simulink library "M160_control_lib"  (Simulink 7.8)
settings: Solver=FixedStepDiscrete  StartTime=0.0  StopTime=10.0  RelTol=1e-3
PreLoadFcn:
  | update_path
undefined symbols (not defined in the file): Egc_tiTEgasFilt, ehooks_medc17flex_devlib_io_block, Fmc_facKFuelMassCorr, Fmc_tiTFuelMassCorr, Itc_rpmEngSpdHyst, Itc_rpmEngSpdMax, Tvc_facDutycyclePIDLimitMax, Tvc_facDutycyclePIDLimitMin, Tvc_facKDutycycle, Tvc_tiTnDutycycle, Tvc_tiTvDutycycle
libraries: simulink x6
(part 1 of 2)
CloseFcn:
  | clear
settings Model: Creator=WLB9FE  LastModifiedBy=Tiger

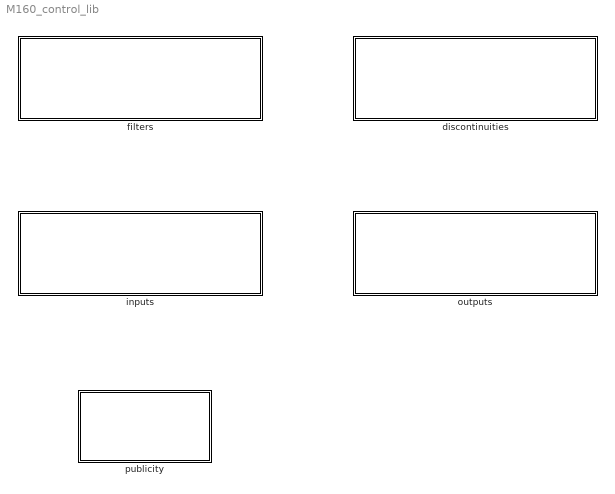
== system M160_control_lib ==
  discontinuities : Subsystem
      mask Display: fprintf('discontinuities')
  filters : Subsystem
      mask Display: fprintf('filters')
  inputs : Subsystem
      mask Display: fprintf('inputs')
  outputs : Subsystem
      mask Display: fprintf('outputs')
  publicity : Subsystem
      mask Description: ETAS
      mask Display: image(imread('ETAS_Logo.jpg'))

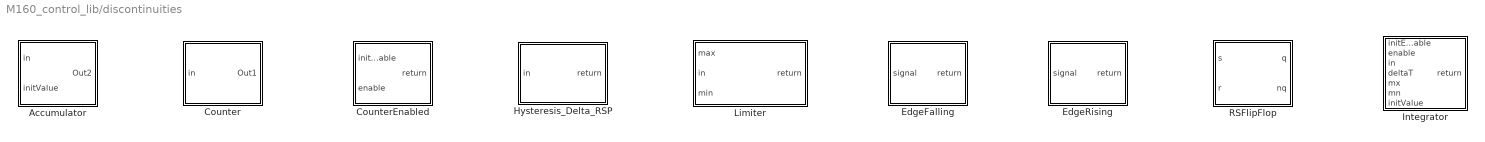
== system M160_control_lib/discontinuities ==
  Accumulator : Subsystem
      mask Description: Accumulator
      mask Display: image(imread('Accumulator.jpg'))
  Counter : Subsystem
      mask Description: Counter
      mask Display: image(imread('Counter.jpg'))
  CounterEnabled : Subsystem
      mask Description: Counter
      mask Display: image(imread('CounterEnabled.jpg'))
  EdgeFalling : Subsystem
      mask Description: EdgeFalling
      mask Display: image(imread('EdgeFalling.jpg'))
  EdgeRising : Subsystem
      mask Description: EdgeRising
      mask Display: image(imread('EdgeRising.jpg'))
  Hysteresis_Delta_RSP : Subsystem
      mask Description: Hysteresis_Delta_RSP
      mask Display: image(imread('HysteresDeltaR.jpg'))
  Integrator : Subsystem
      mask Description: Integrator
      mask Display: image(imread('Integrator.jpg'))
  Limiter : Subsystem
      mask Description: Limiter
      mask Display: image(imread('Limiter.jpg'))
  RSFlipFlop : Subsystem
      mask Description: RSFlipFlop
      mask Display: image(imread('RSFlipFlop.jpg'))

== system M160_control_lib/filters ==
  DT1 : Subsystem
      mask Description: DT1
      mask Display: image(imread('DT1.jpg'))
  DT1_Fcn : Subsystem
      mask Description: DT1_Fcn
      mask Display: image(imread('DT1.jpg'))
  LowpassT : Subsystem
      mask Description: LowpassT
      mask Display: image(imread('LowpassT.jpg'))
  LowpassT_Fcn : Subsystem
      mask Description: LowpassT_Fcn
      mask Display: image(imread('LowpassT.jpg'))
  PID_Limit_AWU : Subsystem
      mask Description: PID_Limit_AWU
      mask Display: image(imread('PID_Limit_AWU.jpg'))
  PID_Limit_AWU_Fcn : Subsystem
      mask Description: PID_Limit_AWU_Fcn
      mask Display: image(imread('PID_Limit_AWU.jpg'))

== system M160_control_lib/inputs ==
  G1_ADC_Input_Receive : Subsystem  LoadFcn=ehooks_medc17flex_devlib_io_block('load');  InitFcn=ehooks_medc17flex_devlib_io_block('init');  StartFcn=ehooks_medc17flex_devlib_io_block('start');  StopFcn=ehooks_medc17flex_devlib_io_block('stop');  ClipboardFcn=ehooks_medc17flex_devlib_io_block('clipboard', 0); % Second argument just needed to indicate null block. See callback handler.  mask{ChannelName=<empty>}
      mask prompts: ChannelName "Channel name"
      mask init:
      | ehooks_medc17flex_devlib_io_block('mask_init');
      settings: AttributesFormatString=Channel name: '%<ChannelName>'  CopyFcn=ehooks_medc17flex_devlib_io_block('copy');  DeleteFcn=ehooks_medc17flex_devlib_io_block('delete');  UndoDeleteFcn=ehooks_medc17flex_devlib_io_block('undo_delete');  ModelCloseFcn=ehooks_medc17flex_devlib_io_block('model_close');  PreSaveFcn=ehooks_medc17flex_devlib_io_block('pre_save');  PostSaveFcn=ehooks_medc17flex_devlib_io_block('post_save');  NameChangeFcn=ehooks_medc17flex_devlib_io_block('name_change');  DestroyFcn=ehooks_medc17flex_devlib_io_block('destroy', 0); % Second argument just needed to indicate null block. See callback handler.  OpenFcn=ehooks_medc17flex_devlib_io_block('open');  CloseFcn=ehooks_medc17flex_devlib_io_block('close');  ParentCloseFcn=ehooks_medc17flex_devlib_io_block('parent_close');  MoveFcn=ehooks_medc17flex_devlib_io_block('move');
      mask StyleString: popup(<empty>|I_A_AN01|I_A_AN02|I_A_AN03|I_A_AN05|I_A_AN06|I_A_AN07|I_A_AN08|I_A_AN10|I_A_AN11|I_A_AN12|I_A_AN13|I_A_AN14|I_A_AN15|I_A_AN16|I_A_AN17|I_A_AN18|I_A_AN19|I_A_AN20|I_A_AN21|I_A_AN23|I_A_AN32|I_A_AN35|I_A_AN36|I_A_AN37|I_A_AN39|I_A_AN100|I_A_AN101|I_A_AN103|I_A_AN104|I_A_AN105|I_A_AN106)
      mask Display: image(imread('Input_Analog.jpg'))
  G1_Digital_Input_Receive : Subsystem  LoadFcn=ehooks_medc17flex_devlib_io_block('load');  InitFcn=ehooks_medc17flex_devlib_io_block('init');  StartFcn=ehooks_medc17flex_devlib_io_block('start');  StopFcn=ehooks_medc17flex_devlib_io_block('stop');  ClipboardFcn=ehooks_medc17flex_devlib_io_block('clipboard', 0); % Second argument just needed to indicate null block. See callback handler.  mask{ChannelName=<empty>}
      mask prompts: ChannelName "Channel name"
      mask init:
      | ehooks_medc17flex_devlib_io_block('mask_init');
      settings: AttributesFormatString=Channel name: '%<ChannelName>'  CopyFcn=ehooks_medc17flex_devlib_io_block('copy');  DeleteFcn=ehooks_medc17flex_devlib_io_block('delete');  UndoDeleteFcn=ehooks_medc17flex_devlib_io_block('undo_delete');  ModelCloseFcn=ehooks_medc17flex_devlib_io_block('model_close');  PreSaveFcn=ehooks_medc17flex_devlib_io_block('pre_save');  PostSaveFcn=ehooks_medc17flex_devlib_io_block('post_save');  NameChangeFcn=ehooks_medc17flex_devlib_io_block('name_change');  DestroyFcn=ehooks_medc17flex_devlib_io_block('destroy', 0); % Second argument just needed to indicate null block. See callback handler.  OpenFcn=ehooks_medc17flex_devlib_io_block('open');  CloseFcn=ehooks_medc17flex_devlib_io_block('close');  ParentCloseFcn=ehooks_medc17flex_devlib_io_block('parent_close');  MoveFcn=ehooks_medc17flex_devlib_io_block('move');
      mask StyleString: popup(<empty>|I_S_T15|I_S_DIG02|I_S_DIG05|I_S_DIG13|I_S_DIG14|I_S_DIG15|I_S_DIG16|I_S_DIG17|I_S_DIG20|I_S_DIG50)
      mask Display: image(imread('Input_Digital.jpg'))
  G1_PWM_Input_Receive : Subsystem  LoadFcn=ehooks_medc17flex_devlib_io_block('load');  InitFcn=ehooks_medc17flex_devlib_io_block('init');  StartFcn=ehooks_medc17flex_devlib_io_block('start');  StopFcn=ehooks_medc17flex_devlib_io_block('stop');  ClipboardFcn=ehooks_medc17flex_devlib_io_block('clipboard', 0); % Second argument just needed to indicate null block. See callback handler.  mask{ChannelName=<empty>}
      mask prompts: ChannelName "Channel name"
      mask init:
      | ehooks_medc17flex_devlib_io_block('mask_init');
      settings: AttributesFormatString=Channel name: '%<ChannelName>'  CopyFcn=ehooks_medc17flex_devlib_io_block('copy');  DeleteFcn=ehooks_medc17flex_devlib_io_block('delete');  UndoDeleteFcn=ehooks_medc17flex_devlib_io_block('undo_delete');  ModelCloseFcn=ehooks_medc17flex_devlib_io_block('model_close');  PreSaveFcn=ehooks_medc17flex_devlib_io_block('pre_save');  PostSaveFcn=ehooks_medc17flex_devlib_io_block('post_save');  NameChangeFcn=ehooks_medc17flex_devlib_io_block('name_change');  DestroyFcn=ehooks_medc17flex_devlib_io_block('destroy', 0); % Second argument just needed to indicate null block. See callback handler.  OpenFcn=ehooks_medc17flex_devlib_io_block('open');  CloseFcn=ehooks_medc17flex_devlib_io_block('close');  ParentCloseFcn=ehooks_medc17flex_devlib_io_block('parent_close');  MoveFcn=ehooks_medc17flex_devlib_io_block('move');
      mask StyleString: popup(<empty>|I_F_DF00|I_F_DF04|I_F_DF06|I_F_DF21|I_F_DF22)
      mask Display: image(imread('Input_Frequency.jpg'))

== system M160_control_lib/outputs ==
  G1_DigOut_Ctrl : Subsystem  LoadFcn=ehooks_medc17flex_devlib_io_block('load');  InitFcn=ehooks_medc17flex_devlib_io_block('init');  StartFcn=ehooks_medc17flex_devlib_io_block('start');  StopFcn=ehooks_medc17flex_devlib_io_block('stop');  ClipboardFcn=ehooks_medc17flex_devlib_io_block('clipboard', 0); % Second argument just needed to indicate null block. See callback handler.  mask{ChannelName=<empty>}
      mask prompts: ChannelName "Channel name"
      mask init:
      | ehooks_medc17flex_devlib_io_block('mask_init');
      settings: AttributesFormatString=Channel name: '%<ChannelName>'  CopyFcn=ehooks_medc17flex_devlib_io_block('copy');  DeleteFcn=ehooks_medc17flex_devlib_io_block('delete');  UndoDeleteFcn=ehooks_medc17flex_devlib_io_block('undo_delete');  ModelCloseFcn=ehooks_medc17flex_devlib_io_block('model_close');  PreSaveFcn=ehooks_medc17flex_devlib_io_block('pre_save');  PostSaveFcn=ehooks_medc17flex_devlib_io_block('post_save');  NameChangeFcn=ehooks_medc17flex_devlib_io_block('name_change');  DestroyFcn=ehooks_medc17flex_devlib_io_block('destroy', 0); % Second argument just needed to indicate null block. See callback handler.  OpenFcn=ehooks_medc17flex_devlib_io_block('open');  CloseFcn=ehooks_medc17flex_devlib_io_block('close');  ParentCloseFcn=ehooks_medc17flex_devlib_io_block('parent_close');  MoveFcn=ehooks_medc17flex_devlib_io_block('move');
      mask StyleString: popup(<empty>|O_S_MRLY|O_S_RL09|O_S_RL14|O_S_RL29|O_S_RL30|O_S_RL31|O_S_RL33|O_S_RL34|O_S_RL35|O_S_RL41|O_S_RL43)
      mask Display: image(imread('Output_Digital.jpg'))
  G1_DigOut_GetError : Subsystem  LoadFcn=ehooks_medc17flex_devlib_io_block('load');  InitFcn=ehooks_medc17flex_devlib_io_block('init');  StartFcn=ehooks_medc17flex_devlib_io_block('start');  StopFcn=ehooks_medc17flex_devlib_io_block('stop');  ClipboardFcn=ehooks_medc17flex_devlib_io_block('clipboard', 0); % Second argument just needed to indicate null block. See callback handler.  mask{ChannelName=<empty>}
      mask prompts: ChannelName "Channel name"
      mask init:
      | ehooks_medc17flex_devlib_io_block('mask_init');
      settings: AttributesFormatString=Channel name: '%<ChannelName>'  CopyFcn=ehooks_medc17flex_devlib_io_block('copy');  DeleteFcn=ehooks_medc17flex_devlib_io_block('delete');  UndoDeleteFcn=ehooks_medc17flex_devlib_io_block('undo_delete');  ModelCloseFcn=ehooks_medc17flex_devlib_io_block('model_close');  PreSaveFcn=ehooks_medc17flex_devlib_io_block('pre_save');  PostSaveFcn=ehooks_medc17flex_devlib_io_block('post_save');  NameChangeFcn=ehooks_medc17flex_devlib_io_block('name_change');  DestroyFcn=ehooks_medc17flex_devlib_io_block('destroy', 0); % Second argument just needed to indicate null block. See callback handler.  OpenFcn=ehooks_medc17flex_devlib_io_block('open');  CloseFcn=ehooks_medc17flex_devlib_io_block('close');  ParentCloseFcn=ehooks_medc17flex_devlib_io_block('parent_close');  MoveFcn=ehooks_medc17flex_devlib_io_block('move');
      mask StyleString: popup(<empty>|O_S_MRLY|O_S_RL09|O_S_RL14|O_S_RL29|O_S_RL30|O_S_RL31|O_S_RL33|O_S_RL34|O_S_RL35|O_S_RL41|O_S_RL43)
      mask Display: image(imread('Output_Digital_Diagnosis.jpg'))
  G1_HbridgeOut_Ctrl : Subsystem  LoadFcn=ehooks_medc17flex_devlib_io_block('load');  InitFcn=ehooks_medc17flex_devlib_io_block('init');  StartFcn=ehooks_medc17flex_devlib_io_block('start');  StopFcn=ehooks_medc17flex_devlib_io_block('stop');  ClipboardFcn=ehooks_medc17flex_devlib_io_block('clipboard', 0); % Second argument just needed to indicate null block. See callback handler.  mask{ChannelName=<empty>}
      mask prompts: ChannelName "Channel name"
      mask init:
      | ehooks_medc17flex_devlib_io_block('mask_init');
      settings: AttributesFormatString=Channel name: '%<ChannelName>'  CopyFcn=ehooks_medc17flex_devlib_io_block('copy');  DeleteFcn=ehooks_medc17flex_devlib_io_block('delete');  UndoDeleteFcn=ehooks_medc17flex_devlib_io_block('undo_delete');  ModelCloseFcn=ehooks_medc17flex_devlib_io_block('model_close');  PreSaveFcn=ehooks_medc17flex_devlib_io_block('pre_save');  PostSaveFcn=ehooks_medc17flex_devlib_io_block('post_save');  NameChangeFcn=ehooks_medc17flex_devlib_io_block('name_change');  DestroyFcn=ehooks_medc17flex_devlib_io_block('destroy', 0); % Second argument just needed to indicate null block. See callback handler.  OpenFcn=ehooks_medc17flex_devlib_io_block('open');  CloseFcn=ehooks_medc17flex_devlib_io_block('close');  ParentCloseFcn=ehooks_medc17flex_devlib_io_block('parent_close');  MoveFcn=ehooks_medc17flex_devlib_io_block('move');
      mask StyleString: popup(<empty>|O_T_DC1|O_T_DC2|O_T_DC3)
      mask Display: image(imread('Output_HBridge.jpg'))
  G1_Hbridge_Get_error : Subsystem  LoadFcn=ehooks_medc17flex_devlib_io_block('load');  InitFcn=ehooks_medc17flex_devlib_io_block('init');  StartFcn=ehooks_medc17flex_devlib_io_block('start');  StopFcn=ehooks_medc17flex_devlib_io_block('stop');  ClipboardFcn=ehooks_medc17flex_devlib_io_block('clipboard', 0); % Second argument just needed to indicate null block. See callback handler.  mask{ChannelName=<empty>}
      mask prompts: ChannelName "Channel name"
      mask init:
      | ehooks_medc17flex_devlib_io_block('mask_init');
      settings: AttributesFormatString=Channel name: '%<ChannelName>'  CopyFcn=ehooks_medc17flex_devlib_io_block('copy');  DeleteFcn=ehooks_medc17flex_devlib_io_block('delete');  UndoDeleteFcn=ehooks_medc17flex_devlib_io_block('undo_delete');  ModelCloseFcn=ehooks_medc17flex_devlib_io_block('model_close');  PreSaveFcn=ehooks_medc17flex_devlib_io_block('pre_save');  PostSaveFcn=ehooks_medc17flex_devlib_io_block('post_save');  NameChangeFcn=ehooks_medc17flex_devlib_io_block('name_change');  DestroyFcn=ehooks_medc17flex_devlib_io_block('destroy', 0); % Second argument just needed to indicate null block. See callback handler.  OpenFcn=ehooks_medc17flex_devlib_io_block('open');  CloseFcn=ehooks_medc17flex_devlib_io_block('close');  ParentCloseFcn=ehooks_medc17flex_devlib_io_block('parent_close');  MoveFcn=ehooks_medc17flex_devlib_io_block('move');
      mask StyleString: popup(<empty>|O_T_DC1|O_T_DC2|O_T_DC3)
      mask Display: image(imread('Output_HBridge_Diagnosis.jpg'))
  G1_IGN_SetParam_for_PFI : Subsystem  LoadFcn=ehooks_medc17flex_devlib_io_block('load');  InitFcn=ehooks_medc17flex_devlib_io_block('init');  StartFcn=ehooks_medc17flex_devlib_io_block('start');  StopFcn=ehooks_medc17flex_devlib_io_block('stop');  ClipboardFcn=ehooks_medc17flex_devlib_io_block('clipboard', 0); % Second argument just needed to indicate null block. See callback handler.  mask{handleName=IGNORED}
      mask prompts: handleName "PlaceHolder_IGNORED"
      mask init:
      | ehooks_medc17flex_devlib_io_block('mask_init');
      settings: CopyFcn=ehooks_medc17flex_devlib_io_block('copy');  DeleteFcn=ehooks_medc17flex_devlib_io_block('delete');  UndoDeleteFcn=ehooks_medc17flex_devlib_io_block('undo_delete');  ModelCloseFcn=ehooks_medc17flex_devlib_io_block('model_close');  PreSaveFcn=ehooks_medc17flex_devlib_io_block('pre_save');  PostSaveFcn=ehooks_medc17flex_devlib_io_block('post_save');  NameChangeFcn=ehooks_medc17flex_devlib_io_block('name_change');  DestroyFcn=ehooks_medc17flex_devlib_io_block('destroy', 0); % Second argument just needed to indicate null block. See callback handler.  OpenFcn=ehooks_medc17flex_devlib_io_block('open');  CloseFcn=ehooks_medc17flex_devlib_io_block('close');  ParentCloseFcn=ehooks_medc17flex_devlib_io_block('parent_close');  MoveFcn=ehooks_medc17flex_devlib_io_block('move');
      mask StyleString: popup(IGNORED)
      mask Display: image(imread('IgnClPfi.jpg'))
  G1_InjVlvPFI_SetParam : Subsystem  LoadFcn=ehooks_medc17flex_devlib_io_block('load');  InitFcn=ehooks_medc17flex_devlib_io_block('init');  StartFcn=ehooks_medc17flex_devlib_io_block('start');  StopFcn=ehooks_medc17flex_devlib_io_block('stop');  ClipboardFcn=ehooks_medc17flex_devlib_io_block('clipboard', 0); % Second argument just needed to indicate null block. See callback handler.  mask{ChannelName=IGNORED}
      mask prompts: ChannelName "PlaceHolder_IGNORED"
      mask init:
      | ehooks_medc17flex_devlib_io_block('mask_init');
      settings: CopyFcn=ehooks_medc17flex_devlib_io_block('copy');  DeleteFcn=ehooks_medc17flex_devlib_io_block('delete');  UndoDeleteFcn=ehooks_medc17flex_devlib_io_block('undo_delete');  ModelCloseFcn=ehooks_medc17flex_devlib_io_block('model_close');  PreSaveFcn=ehooks_medc17flex_devlib_io_block('pre_save');  PostSaveFcn=ehooks_medc17flex_devlib_io_block('post_save');  NameChangeFcn=ehooks_medc17flex_devlib_io_block('name_change');  DestroyFcn=ehooks_medc17flex_devlib_io_block('destroy', 0); % Second argument just needed to indicate null block. See callback handler.  OpenFcn=ehooks_medc17flex_devlib_io_block('open');  CloseFcn=ehooks_medc17flex_devlib_io_block('close');  ParentCloseFcn=ehooks_medc17flex_devlib_io_block('parent_close');  MoveFcn=ehooks_medc17flex_devlib_io_block('move');
      mask StyleString: popup(IGNORED)
      mask Display: image(imread('InjVlvPfi.jpg'))
  G1_Inj_Set_DEVE_forPFI : Subsystem  LoadFcn=ehooks_medc17flex_devlib_io_block('load');  InitFcn=ehooks_medc17flex_devlib_io_block('init');  StartFcn=ehooks_medc17flex_devlib_io_block('start');  StopFcn=ehooks_medc17flex_devlib_io_block('stop');  ClipboardFcn=ehooks_medc17flex_devlib_io_block('clipboard', 0); % Second argument just needed to indicate null block. See callback handler.  mask{ChannelName=IGNORED}
      mask prompts: ChannelName "PlaceHolder_IGNORED"
      mask help: InjVlvDeve
      mask init:
      | ehooks_medc17flex_devlib_io_block('mask_init');
      settings: CopyFcn=ehooks_medc17flex_devlib_io_block('copy');  DeleteFcn=ehooks_medc17flex_devlib_io_block('delete');  UndoDeleteFcn=ehooks_medc17flex_devlib_io_block('undo_delete');  ModelCloseFcn=ehooks_medc17flex_devlib_io_block('model_close');  PreSaveFcn=ehooks_medc17flex_devlib_io_block('pre_save');  PostSaveFcn=ehooks_medc17flex_devlib_io_block('post_save');  NameChangeFcn=ehooks_medc17flex_devlib_io_block('name_change');  DestroyFcn=ehooks_medc17flex_devlib_io_block('destroy', 0); % Second argument just needed to indicate null block. See callback handler.  OpenFcn=ehooks_medc17flex_devlib_io_block('open');  CloseFcn=ehooks_medc17flex_devlib_io_block('close');  ParentCloseFcn=ehooks_medc17flex_devlib_io_block('parent_close');  MoveFcn=ehooks_medc17flex_devlib_io_block('move');
      mask StyleString: popup(IGNORED)
      mask Display: image(imread('InjVlvPfi.jpg'))
  G1_PWM_Output_Ctrl : Subsystem  LoadFcn=ehooks_medc17flex_devlib_io_block('load');  InitFcn=ehooks_medc17flex_devlib_io_block('init');  StartFcn=ehooks_medc17flex_devlib_io_block('start');  StopFcn=ehooks_medc17flex_devlib_io_block('stop');  ClipboardFcn=ehooks_medc17flex_devlib_io_block('clipboard', 0); % Second argument just needed to indicate null block. See callback handler.  mask{ChannelName=<empty>}
      mask prompts: ChannelName "Channel name"
      mask init:
      | ehooks_medc17flex_devlib_io_block('mask_init');
      settings: AttributesFormatString=Channel name: '%<ChannelName>'  CopyFcn=ehooks_medc17flex_devlib_io_block('copy');  DeleteFcn=ehooks_medc17flex_devlib_io_block('delete');  UndoDeleteFcn=ehooks_medc17flex_devlib_io_block('undo_delete');  ModelCloseFcn=ehooks_medc17flex_devlib_io_block('model_close');  PreSaveFcn=ehooks_medc17flex_devlib_io_block('pre_save');  PostSaveFcn=ehooks_medc17flex_devlib_io_block('post_save');  NameChangeFcn=ehooks_medc17flex_devlib_io_block('name_change');  DestroyFcn=ehooks_medc17flex_devlib_io_block('destroy', 0); % Second argument just needed to indicate null block. See callback handler.  OpenFcn=ehooks_medc17flex_devlib_io_block('open');  CloseFcn=ehooks_medc17flex_devlib_io_block('close');  ParentCloseFcn=ehooks_medc17flex_devlib_io_block('parent_close');  MoveFcn=ehooks_medc17flex_devlib_io_block('move');
      mask StyleString: popup(<empty>|O_T_RL10|O_T_RL13|O_T_RL19|O_T_RL20|O_T_RL22|O_T_RL23|O_T_RL25|O_T_RL26|O_T_RL27|O_T_RL28|O_T_RL38|O_T_RL39|O_T_RL40|O_T_RL42|O_T_RL44|O_T_RL45|O_T_RL46|O_T_RL47|O_T_RL48|O_T_RL49|O_T_RL50|O_T_RH02)
      mask Display: image(imread('Output_PWM.jpg'))
  G1_PwmOut_Get_error : Subsystem  LoadFcn=ehooks_medc17flex_devlib_io_block('load');  InitFcn=ehooks_medc17flex_devlib_io_block('init');  StartFcn=ehooks_medc17flex_devlib_io_block('start');  StopFcn=ehooks_medc17flex_devlib_io_block('stop');  ClipboardFcn=ehooks_medc17flex_devlib_io_block('clipboard', 0); % Second argument just needed to indicate null block. See callback handler.  mask{ChannelName=<empty>}
      mask prompts: ChannelName "Channel name"
      mask init:
      | ehooks_medc17flex_devlib_io_block('mask_init');
      settings: AttributesFormatString=Channel name: '%<ChannelName>'  CopyFcn=ehooks_medc17flex_devlib_io_block('copy');  DeleteFcn=ehooks_medc17flex_devlib_io_block('delete');  UndoDeleteFcn=ehooks_medc17flex_devlib_io_block('undo_delete');  ModelCloseFcn=ehooks_medc17flex_devlib_io_block('model_close');  PreSaveFcn=ehooks_medc17flex_devlib_io_block('pre_save');  PostSaveFcn=ehooks_medc17flex_devlib_io_block('post_save');  NameChangeFcn=ehooks_medc17flex_devlib_io_block('name_change');  DestroyFcn=ehooks_medc17flex_devlib_io_block('destroy', 0); % Second argument just needed to indicate null block. See callback handler.  OpenFcn=ehooks_medc17flex_devlib_io_block('open');  CloseFcn=ehooks_medc17flex_devlib_io_block('close');  ParentCloseFcn=ehooks_medc17flex_devlib_io_block('parent_close');  MoveFcn=ehooks_medc17flex_devlib_io_block('move');
      mask StyleString: popup(<empty>|O_T_RL10|O_T_RL13|O_T_RL19|O_T_RL20|O_T_RL22|O_T_RL23|O_T_RL25|O_T_RL26|O_T_RL27|O_T_RL28|O_T_RL38|O_T_RL39|O_T_RL40|O_T_RL42|O_T_RL44|O_T_RL45|O_T_RL46|O_T_RL47|O_T_RL48|O_T_RL49|O_T_RL50|O_T_RH02)
      mask Display: image(imread('Output_PWM_Diagnosis.jpg'))

== system M160_control_lib/publicity ==

== system M160_control_lib/discontinuities/Accumulator ==
  in : Inport
  initValue : Inport  Port=2
  Add : Sum
  MATLAB Function : MATLAB Function  TreatAsAtomicUnit=on
  Switch2 : Switch  Threshold=1
  Unit Delay : UnitDelay  SampleTime=-1
  Out2 : Outport
  wires:
  in/1 -> Add/1, MATLAB Function/1(u)
  Unit Delay/1 -> Add/2
  Switch2/1 -> Out2/1
  initValue/1 -> Switch2/3
  Add/1 -> Switch2/1, Unit Delay/1
  MATLAB Function/1(y) -> Switch2/2

== system M160_control_lib/discontinuities/Counter ==
  in : Inport
  Add1 : Sum
  Constant1 : Constant  OutDataTypeStr=single
  Constant2 : Constant  Value=0  OutDataTypeStr=single
  MATLAB Function : MATLAB Function  TreatAsAtomicUnit=on
  Switch2 : Switch  Threshold=1
  Unit Delay1 : UnitDelay  SampleTime=-1
  Out1 : Outport
  wires:
  Constant1/1 -> Add1/1
  Unit Delay1/1 -> Add1/2
  Switch2/1 -> Out1/1
  Constant2/1 -> Switch2/3
  Add1/1 -> Switch2/1, Unit Delay1/1
  MATLAB Function/1(y) -> Switch2/2
  in/1 -> MATLAB Function/1(u)

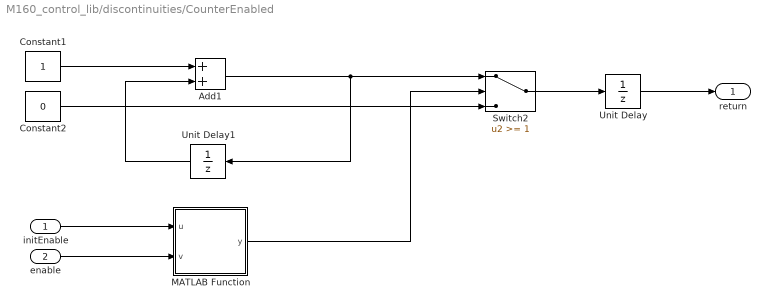
== system M160_control_lib/discontinuities/CounterEnabled ==
  initEnable : Inport
  enable : Inport  Port=2
  Add1 : Sum
  Constant1 : Constant  OutDataTypeStr=single
  Constant2 : Constant  Value=0  OutDataTypeStr=single
  MATLAB Function : MATLAB Function  TreatAsAtomicUnit=on
  Switch2 : Switch  Threshold=1
  Unit Delay : UnitDelay  SampleTime=-1
  Unit Delay1 : UnitDelay  SampleTime=-1
  return : Outport
  wires:
  initEnable/1 -> MATLAB Function/1(u)
  MATLAB Function/1(y) -> Switch2/2
  Add1/1 -> Unit Delay1/1, Switch2/1
  Constant2/1 -> Switch2/3
  Switch2/1 -> Unit Delay/1
  Unit Delay1/1 -> Add1/2
  Constant1/1 -> Add1/1
  enable/1 -> MATLAB Function/2(v)
  Unit Delay/1 -> return/1

== system M160_control_lib/discontinuities/EdgeFalling ==
  signal : Inport
  Detect Decrease : simulink/Logic and Bit Operations/Detect Decrease  vinit=0.0  InputProcessing=Inherited  OutDataTypeStr=boolean
  return : Outport
  wires:
  Detect Decrease/1 -> return/1
  signal/1 -> Detect Decrease/1

== system M160_control_lib/discontinuities/EdgeRising ==
  signal : Inport
  Detect Increase : simulink/Logic and Bit Operations/Detect Increase  vinit=0.0  InputProcessing=Inherited  OutDataTypeStr=boolean
  return : Outport
  wires:
  Detect Increase/1 -> return/1
  signal/1 -> Detect Increase/1

== system M160_control_lib/discontinuities/Hysteresis_Delta_RSP ==
  in : Inport
  Relay : Relay  OnSwitchValue=Itc_rpmEngSpdMax  OffSwitchValue=Itc_rpmEngSpdMax-Itc_rpmEngSpdHyst  OutDataTypeStr=Inherit: Inherit via back propagation
  return : Outport
  wires:
  Relay/1 -> return/1
  in/1 -> Relay/1

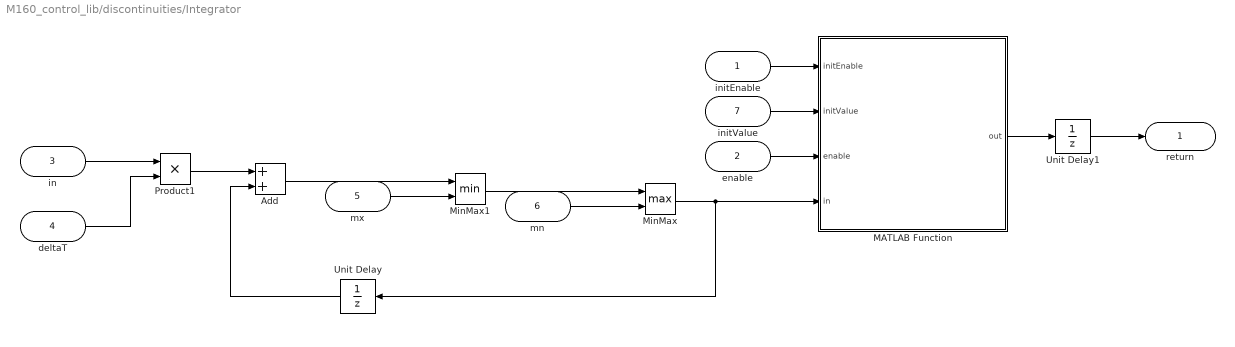
== system M160_control_lib/discontinuities/Integrator ==
  initEnable : Inport
  enable : Inport  Port=2
  in : Inport  Port=3
  deltaT : Inport  Port=4
  mx : Inport  Port=5
  mn : Inport  Port=6
  initValue : Inport  Port=7
  Add : Sum
  MATLAB Function : MATLAB Function  TreatAsAtomicUnit=on
  MinMax : MinMax  Function=max  Inputs=2
  MinMax1 : MinMax  Inputs=2
  Product1 : Product  OutDataTypeStr=Inherit: Same as first input
  Unit Delay : UnitDelay  SampleTime=-1
  Unit Delay1 : UnitDelay  SampleTime=-1
  return : Outport
  wires:
  deltaT/1 -> Product1/2
  in/1 -> Product1/1
  Product1/1 -> Add/1
  Add/1 -> MinMax1/1
  mx/1 -> MinMax1/2
  MinMax1/1 -> MinMax/1
  mn/1 -> MinMax/2
  Unit Delay/1 -> Add/2
  MinMax/1 -> Unit Delay/1, MATLAB Function/4(in)
  MATLAB Function/1(out) -> Unit Delay1/1
  enable/1 -> MATLAB Function/3(enable)
  initValue/1 -> MATLAB Function/2(initValue)
  initEnable/1 -> MATLAB Function/1(initEnable)
  Unit Delay1/1 -> return/1

== system M160_control_lib/discontinuities/Limiter ==
  max : Inport
  in : Inport  Port=2
  min : Inport  Port=3
  Saturation Dynamic : simulink/Discontinuities/Saturation Dynamic  OutMin=[]  OutMax=[]  OutDataTypeStr=Inherit: Same as second input  OutDataType=fixdt(1, 16)  OutScaling=2^-10  DoSatur=off
  return : Outport
  wires:
  max/1 -> Saturation Dynamic/1
  in/1 -> Saturation Dynamic/2
  min/1 -> Saturation Dynamic/3
  Saturation Dynamic/1 -> return/1

== system M160_control_lib/discontinuities/RSFlipFlop ==
  s : Inport
  r : Inport  Port=2
  Gain : Gain  OutDataTypeStr=Inherit: Same as input
  Logical Operator3 : Logic  Operator=NOT  AllPortsSameDT=off  OutDataTypeStr=boolean
  MATLAB Function : MATLAB Function  TreatAsAtomicUnit=on
  Unit Delay : UnitDelay  SampleTime=-1
  q : Outport
  nq : Outport  Port=2
  wires:
  Logical Operator3/1 -> nq/1
  r/1 -> MATLAB Function/1(r)
  s/1 -> MATLAB Function/2(s)
  MATLAB Function/1(q) -> Unit Delay/1
  Gain/1 -> q/1
  Unit Delay/1 -> Logical Operator3/1, Gain/1

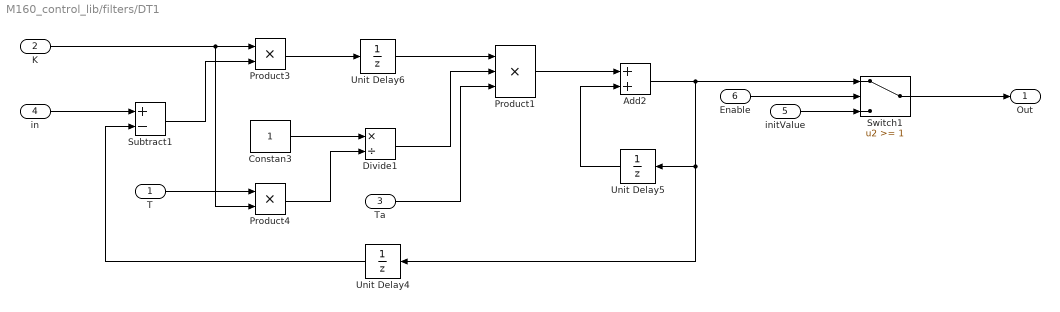
== system M160_control_lib/filters/DT1 ==
  T : Inport
  K : Inport  Port=2
  Ta : Inport  Port=3
  in : Inport  Port=4
  initValue : Inport  Port=5
  Enable : Inport  Port=6
  Add2 : Sum  OutDataTypeStr=Inherit: Same as first input
  Constan3 : Constant  OutDataTypeStr=single
  Divide1 : Product  Inputs=*/  OutDataTypeStr=Inherit: Same as first input
  Product1 : Product  Inputs=3  OutDataTypeStr=Inherit: Same as first input
  Product3 : Product  OutDataTypeStr=Inherit: Same as first input
  Product4 : Product  OutDataTypeStr=Inherit: Same as first input
  Subtract1 : Sum  Inputs=+-
  Switch1 : Switch  Threshold=1
  Unit Delay4 : UnitDelay  SampleTime=-1
  Unit Delay5 : UnitDelay  SampleTime=-1
  Unit Delay6 : UnitDelay  SampleTime=-1
  Out : Outport
  wires:
  initValue/1 -> Switch1/3
  Switch1/1 -> Out/1
  in/1 -> Subtract1/1
  Subtract1/1 -> Product3/2
  K/1 -> Product3/1, Product4/2
  Product3/1 -> Unit Delay6/1
  Unit Delay6/1 -> Product1/1
  Constan3/1 -> Divide1/1
  T/1 -> Product4/1
  Product4/1 -> Divide1/2
  Divide1/1 -> Product1/2
  Product1/1 -> Add2/1
  Add2/1 -> Unit Delay5/1, Unit Delay4/1, Switch1/1
  Unit Delay5/1 -> Add2/2
  Unit Delay4/1 -> Subtract1/2
  Ta/1 -> Product1/3
  Enable/1 -> Switch1/2

== system M160_control_lib/filters/DT1_Fcn ==
  In : Inport
  initValue : Inport  Port=2
  Enable : Inport  Port=3
  Discrete Transfer Fcn : DiscreteTransferFcn  Numerator=[Fmc_facKFuelMassCorr Fmc_facKFuelMassCorr*(0.001/Fmc_tiTFuelMassCorr-1)]  Denominator=[1 -1]  SampleTime=-1  OutDataTypeStr=Inherit: Same as input
  Switch1 : Switch  Threshold=1
  Out : Outport
  wires:
  In/1 -> Discrete Transfer Fcn/1
  initValue/1 -> Switch1/3
  Switch1/1 -> Out/1
  Discrete Transfer Fcn/1 -> Switch1/1
  Enable/1 -> Switch1/2

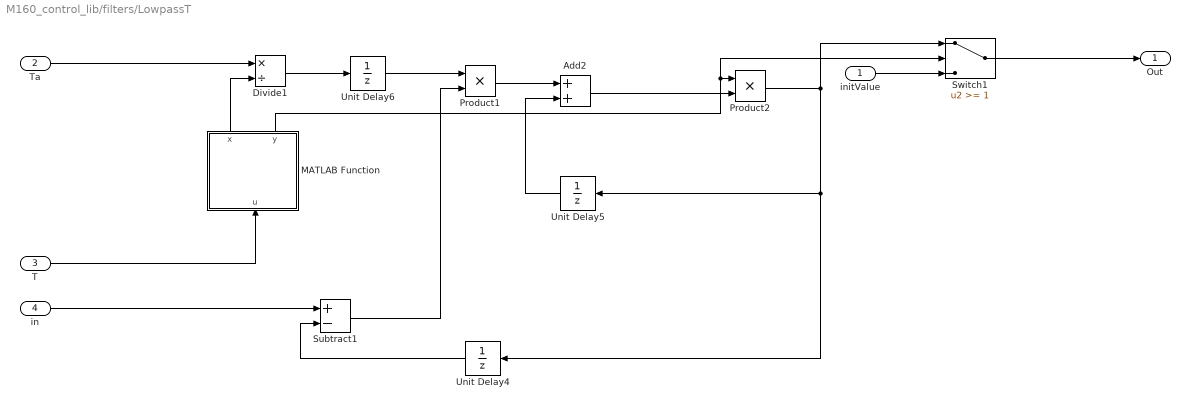
== system M160_control_lib/filters/LowpassT ==
  initValue : Inport
  Ta : Inport  Port=2
  T : Inport  Port=3
  in : Inport  Port=4
  Add2 : Sum  OutDataTypeStr=Inherit: Same as first input
  Divide1 : Product  Inputs=*/  OutDataTypeStr=Inherit: Same as first input
  MATLAB Function : MATLAB Function  TreatAsAtomicUnit=on
  Product1 : Product  OutDataTypeStr=Inherit: Same as first input
  Product2 : Product  OutDataTypeStr=single
  Subtract1 : Sum  Inputs=+-
  Switch1 : Switch  Threshold=1
  Unit Delay4 : UnitDelay  SampleTime=-1
  Unit Delay5 : UnitDelay  SampleTime=-1
  Unit Delay6 : UnitDelay  SampleTime=-1
  Out : Outport
  wires:
  initValue/1 -> Switch1/3
  Switch1/1 -> Out/1
  MATLAB Function/1(x) -> Divide1/2
  MATLAB Function/2(y) -> Switch1/2, Product2/1
  Ta/1 -> Divide1/1
  T/1 -> MATLAB Function/1(u)
  Divide1/1 -> Unit Delay6/1
  Subtract1/1 -> Product1/2
  Product1/1 -> Add2/1
  Unit Delay5/1 -> Add2/2
  Unit Delay6/1 -> Product1/1
  Unit Delay4/1 -> Subtract1/2
  in/1 -> Subtract1/1
  Product2/1 -> Switch1/1, Unit Delay4/1, Unit Delay5/1
  Add2/1 -> Product2/2

== system M160_control_lib/filters/LowpassT_Fcn ==
  initValue : Inport
  In : Inport  Port=2
  T : Inport  Port=3
  Discrete Transfer Fcn : DiscreteTransferFcn  Denominator=[Egc_tiTEgasFilt/0.01 1-Egc_tiTEgasFilt/0.01]  SampleTime=-1  OutDataTypeStr=Inherit: Same as input
  MATLAB Function : MATLAB Function  TreatAsAtomicUnit=on
  Product1 : Product  OutDataTypeStr=single
  Switch1 : Switch  Threshold=1
  Out : Outport
  wires:
  MATLAB Function/1(y) -> Switch1/2, Product1/1
  T/1 -> MATLAB Function/1(u)
  initValue/1 -> Switch1/3
  Switch1/1 -> Out/1
  Product1/1 -> Switch1/1
  Discrete Transfer Fcn/1 -> Product1/2
  In/1 -> Discrete Transfer Fcn/1

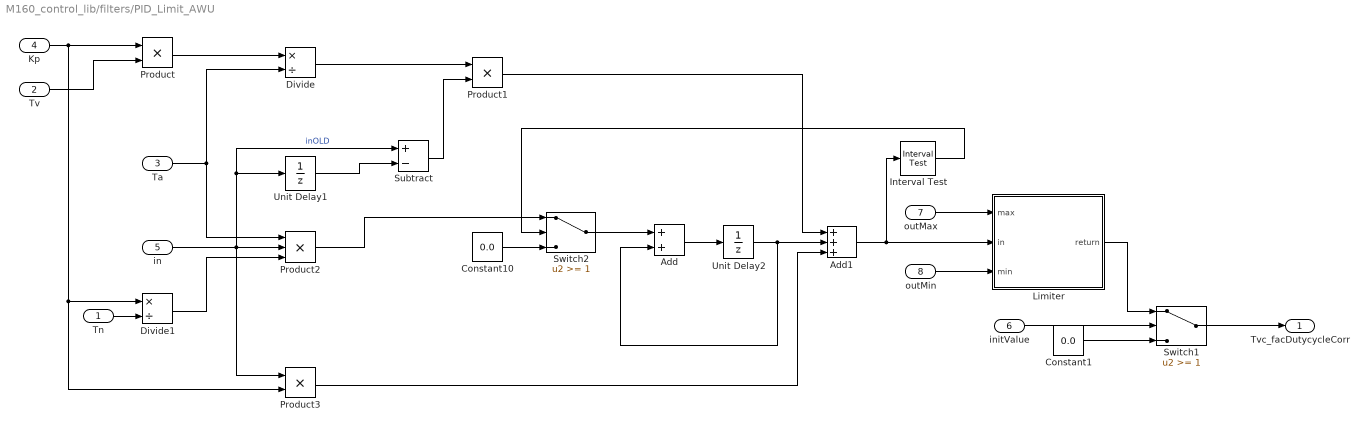
== system M160_control_lib/filters/PID_Limit_AWU ==
  Tn : Inport
  Tv : Inport  Port=2
  Ta : Inport  Port=3
  Kp : Inport  Port=4
  in : Inport  Port=5
  initValue : Inport  Port=6
  outMax : Inport  Port=7
  outMin : Inport  Port=8
  Add : Sum  OutDataTypeStr=Inherit: Same as first input
  Add1 : Sum  Inputs=+++  OutDataTypeStr=Inherit: Same as first input
  Constant1 : Constant  Value=0.0  OutDataTypeStr=single
  Constant10 : Constant  Value=0.0  OutDataTypeStr=single
  Divide : Product  Inputs=*/  OutDataTypeStr=Inherit: Same as first input
  Divide1 : Product  Inputs=*/  OutDataTypeStr=Inherit: Same as first input
  Interval Test : simulink/Logic and Bit Operations/Interval Test  IntervalClosedRight=on  uplimit=Tvc_facDutycyclePIDLimitMax  IntervalClosedLeft=on  lowlimit=Tvc_facDutycyclePIDLimitMin  OutDataTypeStr=boolean
  Limiter : Subsystem
      mask Description: Limiter
      mask Display: image(imread('Limiter.jpg'))
  Product : Product  OutDataTypeStr=Inherit: Same as first input
  Product1 : Product  OutDataTypeStr=Inherit: Same as first input
  Product2 : Product  Inputs=3  OutDataTypeStr=Inherit: Same as first input
  Product3 : Product  OutDataTypeStr=Inherit: Same as first input
  Subtract : Sum  Inputs=+-  OutDataTypeStr=Inherit: Same as first input
  Switch1 : Switch  Threshold=1
  Switch2 : Switch  Threshold=1
  Unit Delay1 : UnitDelay  SampleTime=-1
  Unit Delay2 : UnitDelay  SampleTime=-1
  Tvc_facDutycycleCorr : Outport
  wires:
  Constant10/1 -> Switch2/3
  Product2/1 -> Switch2/1
  Interval Test/1 -> Switch2/2
  Unit Delay2/1 -> Add/2, Add1/2
  Add/1 -> Unit Delay2/1
  Unit Delay1/1 -> Subtract/2
  Kp/1 -> Product/1, Product3/2, Divide1/1
  Tv/1 -> Product/2
  Product/1 -> Divide/1
  Ta/1 -> Product2/1, Divide/2
  Divide/1 -> Product1/1
  Tn/1 -> Divide1/2
  in/1 -> Product2/2, Product3/1, Subtract/1, Unit Delay1/1  "inOLD"
  Divide1/1 -> Product2/3
  Subtract/1 -> Product1/2
  Switch2/1 -> Add/1
  Product3/1 -> Add1/3
  Product1/1 -> Add1/1
  Add1/1 -> Limiter/2(in), Interval Test/1
  outMin/1 -> Limiter/3(min)
  outMax/1 -> Limiter/1(max)
  Constant1/1 -> Switch1/3
  initValue/1 -> Switch1/2
  Switch1/1 -> Tvc_facDutycycleCorr/1
  Limiter/1(return) -> Switch1/1

== system M160_control_lib/filters/PID_Limit_AWU_Fcn ==
  in : Inport
  initValue : Inport  Port=2
  Constant1 : Constant  Value=0.0  OutDataTypeStr=single
  Discrete PID Controller : simulink/Continuous/PID Controller  Controller=PID  TimeDomain=Discrete-time  SampleTime=-1  IntegratorMethod=Forward Euler  FilterMethod=Forward Euler  Form=Parallel  P=Tvc_facKDutycycle  I=Tvc_facKDutycycle/Tvc_tiTnDutycycle  D=Tvc_facKDutycycle*Tvc_tiTvDutycycle  N=Tvc_facKDutycycle*Tvc_tiTvDutycycle/0.01  InitialConditionSource=internal  InitialConditionForIntegrator=0  InitialConditionForFilter=0  ExternalReset=none  LimitOutput=on  UpperSaturationLimit=Tvc_facDutycyclePIDLimitMax  LowerSaturationLimit=Tvc_facDutycyclePIDLimitMin  LinearizeAsGain=off  AntiWindupMode=none  Kb=1  TrackingMode=off  Kt=1  PParamMin=[]  PParamMax=[]  IParamMin=[]  IParamMax=[]  DParamMin=[]  DParamMax=[]  NParamMin=[]  NParamMax=[]  KbParamMin=[]  KbParamMax=[]  KtParamMin=[]  KtParamMax=[]  POutMin=[]  POutMax=[]  IOutMin=[]  IOutMax=[]  DOutMin=[]  DOutMax=[]  NOutMin=[]  NOutMax=[]  KbOutMin=[]  KbOutMax=[]  KtOutMin=[]  KtOutMax=[]  IntegratorOutMin=[]  IntegratorOutMax=[]  FilterOutMin=[]  FilterOutMax=[]  SumOutMin=[]  SumOutMax=[]  SumI1OutMin=[]  SumI1OutMax=[]  SumI2OutMin=[]  SumI2OutMax=[]  SumI3OutMin=[]  SumI3OutMax=[]  SumDOutMin=[]  SumDOutMax=[]  SaturationOutMin=[]  SaturationOutMax=[]  IntegratorContinuousStateAttributes=''  IntegratorStateMustResolveToSignalObject=off  IntegratorRTWStateStorageClass=Auto  FilterContinuousStateAttributes=''  FilterStateMustResolveToSignalObject=off  FilterRTWStateStorageClass=Auto
  Switch1 : Switch  Threshold=1
  Tvc_facDutycycleCorr : Outport
  wires:
  Switch1/1 -> Tvc_facDutycycleCorr/1
  initValue/1 -> Switch1/2
  Constant1/1 -> Switch1/3
  in/1 -> Discrete PID Controller/1  "inOLD"
  Discrete PID Controller/1 -> Switch1/1

== system M160_control_lib/inputs/G1_ADC_Input_Receive ==
  Data Type Conversion2 : DataTypeConversion  OutMin=0.0  OutMax=5.0  OutDataTypeStr=single
  Data Type Conversion3 : DataTypeConversion  OutMin=0.0  OutMax=1.0  OutDataTypeStr=boolean
  FlexECU_DevLib_FcnAPI_Wrapper_SFcn : S-Function  FunctionName=ehooks_medc17flex_devlib_basic_io_fcncall  Parameters=NoInputPorts, NoOutputPorts, InputPortDataTypes, OutputPortDataTypes, CFunctionArgTypes, CFunctionName, ChannelName  EnableBusSupport=off  mask{NoInputPorts=0, NoOutputPorts=2, InputPortDataTypes=, OutputPortDataTypes=uint8,int16, CFunctionArgTypes=ret,ref, CFunctionName=DevLib_Adc_Get, ChannelName=<empty>}
      mask prompts: NoInputPorts "Number of input ports"; NoOutputPorts "Number of output ports"; InputPortDataTypes "Input port data types"; OutputPortDataTypes "Output port data types"; CFunctionArgTypes "C function argument types"; CFunctionName "C function name"; ChannelName "Channel (pin) name"
      mask Display: disp('EHOOKS FlexECU\nDevLib Wrapper\nS-Function')
  Gain : Gain  Gain=5/1023  OutDataTypeStr=Inherit: Same as input
  status : Outport
  uRaw : Outport  Port=2
  wires:
  FlexECU_DevLib_FcnAPI_Wrapper_SFcn/2 -> Data Type Conversion2/1
  FlexECU_DevLib_FcnAPI_Wrapper_SFcn/1 -> Data Type Conversion3/1
  Data Type Conversion3/1 -> status/1
  Data Type Conversion2/1 -> Gain/1
  Gain/1 -> uRaw/1

== system M160_control_lib/inputs/G1_Digital_Input_Receive ==
  Data Type Conversion2 : DataTypeConversion  OutMin=0.0  OutMax=1.0  OutDataTypeStr=boolean
  Data Type Conversion3 : DataTypeConversion  OutMin=0.0  OutMax=1.0  OutDataTypeStr=boolean
  FlexECU_DevLib_FcnAPI_Wrapper_SFcn : S-Function  FunctionName=ehooks_medc17flex_devlib_basic_io_fcncall  Parameters=NoInputPorts, NoOutputPorts, InputPortDataTypes, OutputPortDataTypes, CFunctionArgTypes, CFunctionName, ChannelName  EnableBusSupport=off  mask{NoInputPorts=0, NoOutputPorts=2, InputPortDataTypes=, OutputPortDataTypes=uint8,uint8, CFunctionArgTypes=ret,ref, CFunctionName=DevLib_Dio_Get, ChannelName=<empty>}
      mask prompts: NoInputPorts "Number of input ports"; NoOutputPorts "Number of output ports"; InputPortDataTypes "Input port data types"; OutputPortDataTypes "Output port data types"; CFunctionArgTypes "C function argument types"; CFunctionName "C function name"; ChannelName "Channel (pin) name"
      mask Display: disp('EHOOKS FlexECU\nDevLib Wrapper\nS-Function')
  status : Outport
  stRaw1 : Outport  Port=2
  wires:
  Data Type Conversion2/1 -> stRaw1/1
  Data Type Conversion3/1 -> status/1
  FlexECU_DevLib_FcnAPI_Wrapper_SFcn/1 -> Data Type Conversion3/1
  FlexECU_DevLib_FcnAPI_Wrapper_SFcn/2 -> Data Type Conversion2/1

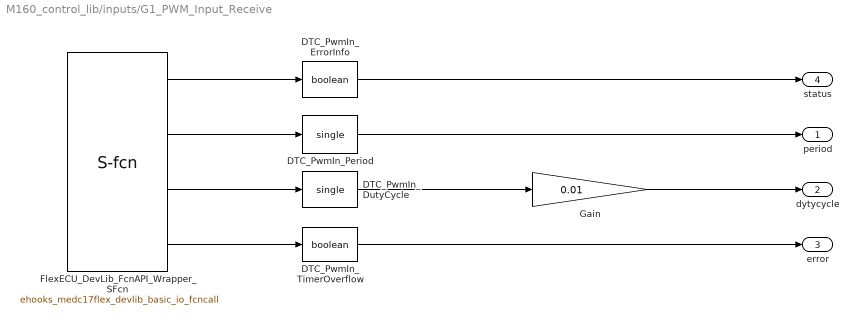
== system M160_control_lib/inputs/G1_PWM_Input_Receive ==
  DTC_PwmIn_DutyCycle : DataTypeConversion  OutDataTypeStr=single
  DTC_PwmIn_ErrorInfo : DataTypeConversion  OutDataTypeStr=boolean
  DTC_PwmIn_Period : DataTypeConversion  OutDataTypeStr=single
  DTC_PwmIn_TimerOverflow : DataTypeConversion  OutDataTypeStr=boolean
  FlexECU_DevLib_FcnAPI_Wrapper_SFcn : S-Function  FunctionName=ehooks_medc17flex_devlib_basic_io_fcncall  Parameters=NoInputPorts, NoOutputPorts, InputPortDataTypes, OutputPortDataTypes, CFunctionArgTypes, CFunctionName, ChannelName  EnableBusSupport=off  mask{NoInputPorts=0, NoOutputPorts=4, InputPortDataTypes=, OutputPortDataTypes=uint8,int32,uint32,uint8, CFunctionArgTypes=ret,ref,ref,ref, CFunctionName=DevLib_Pwm_In, ChannelName=<empty>}
      mask prompts: NoInputPorts "Number of input ports"; NoOutputPorts "Number of output ports"; InputPortDataTypes "Input port data types"; OutputPortDataTypes "Output port data types"; CFunctionArgTypes "C function argument types"; CFunctionName "C function name"; ChannelName "Channel (pin) name"
      mask Display: disp('EHOOKS FlexECU\nDevLib Wrapper\nS-Function')
  Gain : Gain  Gain=0.01
  period : Outport
  dytycycle : Outport  Port=2
  error : Outport  Port=3
  status : Outport  Port=4
  wires:
  DTC_PwmIn_Period/1 -> period/1
  Gain/1 -> dytycycle/1
  DTC_PwmIn_DutyCycle/1 -> Gain/1
  FlexECU_DevLib_FcnAPI_Wrapper_SFcn/4 -> DTC_PwmIn_TimerOverflow/1
  DTC_PwmIn_TimerOverflow/1 -> error/1
  FlexECU_DevLib_FcnAPI_Wrapper_SFcn/3 -> DTC_PwmIn_DutyCycle/1
  FlexECU_DevLib_FcnAPI_Wrapper_SFcn/2 -> DTC_PwmIn_Period/1
  FlexECU_DevLib_FcnAPI_Wrapper_SFcn/1 -> DTC_PwmIn_ErrorInfo/1
  DTC_PwmIn_ErrorInfo/1 -> status/1

== system M160_control_lib/outputs/G1_DigOut_Ctrl ==
  state : Inport
  DTC_DigOut_ctrl : DataTypeConversion  OutDataTypeStr=uint8  RndMeth=Nearest
  DTC_Out1 : DataTypeConversion  OutDataTypeStr=boolean
  FlexECU_DevLib_FcnAPI_Wrapper_SFcn : S-Function  FunctionName=ehooks_medc17flex_devlib_basic_io_fcncall  Parameters=NoInputPorts, NoOutputPorts, InputPortDataTypes, OutputPortDataTypes, CFunctionArgTypes, CFunctionName, ChannelName  EnableBusSupport=off  mask{NoInputPorts=1, NoOutputPorts=1, InputPortDataTypes=uint8, OutputPortDataTypes=uint8, CFunctionArgTypes=ret,val, CFunctionName=DevLib_Dio_Set, ChannelName=<empty>}
      mask prompts: NoInputPorts "Number of input ports"; NoOutputPorts "Number of output ports"; InputPortDataTypes "Input port data types"; OutputPortDataTypes "Output port data types"; CFunctionArgTypes "C function argument types"; CFunctionName "C function name"; ChannelName "Channel (pin) name"
      mask Display: disp('EHOOKS FlexECU\nDevLib Wrapper\nS-Function')
  status : Outport
  wires:
  DTC_DigOut_ctrl/1 -> FlexECU_DevLib_FcnAPI_Wrapper_SFcn/1
  state/1 -> DTC_DigOut_ctrl/1
  FlexECU_DevLib_FcnAPI_Wrapper_SFcn/1 -> DTC_Out1/1
  DTC_Out1/1 -> status/1

== system M160_control_lib/outputs/G1_DigOut_GetError ==
  DTC_DigOut_GetError : DataTypeConversion  OutDataTypeStr=single
  FlexECU_DevLib_FcnAPI_Wrapper_SFcn : S-Function  FunctionName=ehooks_medc17flex_devlib_basic_io_fcncall  Parameters=NoInputPorts, NoOutputPorts, InputPortDataTypes, OutputPortDataTypes, CFunctionArgTypes, CFunctionName, ChannelName  EnableBusSupport=off  mask{NoInputPorts=0, NoOutputPorts=1, InputPortDataTypes=, OutputPortDataTypes=uint8, CFunctionArgTypes=ret, CFunctionName=DevLib_DioSet_GetError, ChannelName=<empty>}
      mask prompts: NoInputPorts "Number of input ports"; NoOutputPorts "Number of output ports"; InputPortDataTypes "Input port data types"; OutputPortDataTypes "Output port data types"; CFunctionArgTypes "C function argument types"; CFunctionName "C function name"; ChannelName "Channel (pin) name"
      mask Display: disp('EHOOKS FlexECU\nDevLib Wrapper\nS-Function')
  status : Outport
  wires:
  DTC_DigOut_GetError/1 -> status/1
  FlexECU_DevLib_FcnAPI_Wrapper_SFcn/1 -> DTC_DigOut_GetError/1

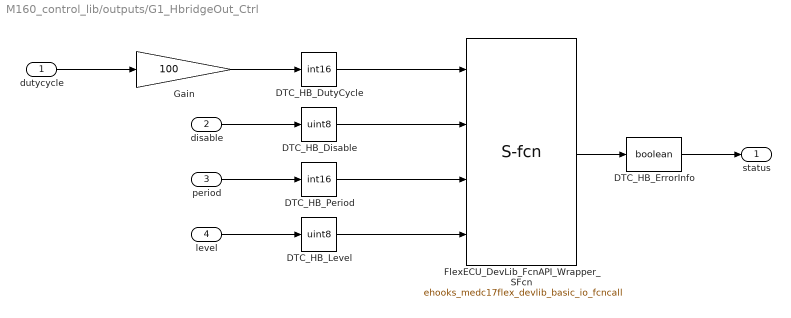
== system M160_control_lib/outputs/G1_HbridgeOut_Ctrl ==
  dutycycle : Inport
  disable : Inport  Port=2
  period : Inport  Port=3
  level : Inport  Port=4
  DTC_HB_Disable : DataTypeConversion  OutDataTypeStr=uint8  RndMeth=Nearest
  DTC_HB_DutyCycle : DataTypeConversion  OutDataTypeStr=int16  RndMeth=Nearest
  DTC_HB_ErrorInfo : DataTypeConversion  OutMin=0.0  OutMax=1.0  OutDataTypeStr=boolean
  DTC_HB_Level : DataTypeConversion  OutDataTypeStr=uint8  RndMeth=Nearest
  DTC_HB_Period : DataTypeConversion  OutDataTypeStr=int16  RndMeth=Nearest
  FlexECU_DevLib_FcnAPI_Wrapper_SFcn : S-Function  FunctionName=ehooks_medc17flex_devlib_basic_io_fcncall  Parameters=NoInputPorts, NoOutputPorts, InputPortDataTypes, OutputPortDataTypes, CFunctionArgTypes, CFunctionName, ChannelName  EnableBusSupport=off  mask{NoInputPorts=4, NoOutputPorts=1, InputPortDataTypes=int16,uint8,int16,uint8, OutputPortDataTypes=uint8, CFunctionArgTypes=ret,val,val,val, val, CFunctionName=DevLib_HBridge_Out, ChannelName=<empty>}
      mask prompts: NoInputPorts "Number of input ports"; NoOutputPorts "Number of output ports"; InputPortDataTypes "Input port data types"; OutputPortDataTypes "Output port data types"; CFunctionArgTypes "C function argument types"; CFunctionName "C function name"; ChannelName "Channel (pin) name"
      mask Display: disp('EHOOKS FlexECU\nDevLib Wrapper\nS-Function')
  Gain : Gain  Gain=100
  status : Outport
  wires:
  dutycycle/1 -> Gain/1
  FlexECU_DevLib_FcnAPI_Wrapper_SFcn/1 -> DTC_HB_ErrorInfo/1
  period/1 -> DTC_HB_Period/1
  level/1 -> DTC_HB_Level/1
  DTC_HB_DutyCycle/1 -> FlexECU_DevLib_FcnAPI_Wrapper_SFcn/1
  DTC_HB_ErrorInfo/1 -> status/1
  DTC_HB_Period/1 -> FlexECU_DevLib_FcnAPI_Wrapper_SFcn/3
  DTC_HB_Level/1 -> FlexECU_DevLib_FcnAPI_Wrapper_SFcn/4
  DTC_HB_Disable/1 -> FlexECU_DevLib_FcnAPI_Wrapper_SFcn/2
  disable/1 -> DTC_HB_Disable/1
  Gain/1 -> DTC_HB_DutyCycle/1

== system M160_control_lib/outputs/G1_Hbridge_Get_error ==
  DTC_HB_GetError : DataTypeConversion  OutMin=0  OutMax=7  OutDataTypeStr=single
  FlexECU_DevLib_FcnAPI_Wrapper_SFcn : S-Function  FunctionName=ehooks_medc17flex_devlib_basic_io_fcncall  Parameters=NoInputPorts, NoOutputPorts, InputPortDataTypes, OutputPortDataTypes, CFunctionArgTypes, CFunctionName, ChannelName  EnableBusSupport=off  mask{NoInputPorts=0, NoOutputPorts=1, InputPortDataTypes=, OutputPortDataTypes=uint8, CFunctionArgTypes=ret, CFunctionName=DevLib_HBridge_GetError, ChannelName=<empty>}
      mask prompts: NoInputPorts "Number of input ports"; NoOutputPorts "Number of output ports"; InputPortDataTypes "Input port data types"; OutputPortDataTypes "Output port data types"; CFunctionArgTypes "C function argument types"; CFunctionName "C function name"; ChannelName "Channel (pin) name"
      mask Display: disp('EHOOKS FlexECU\nDevLib Wrapper\nS-Function')
  status : Outport
  wires:
  DTC_HB_GetError/1 -> status/1
  FlexECU_DevLib_FcnAPI_Wrapper_SFcn/1 -> DTC_HB_GetError/1

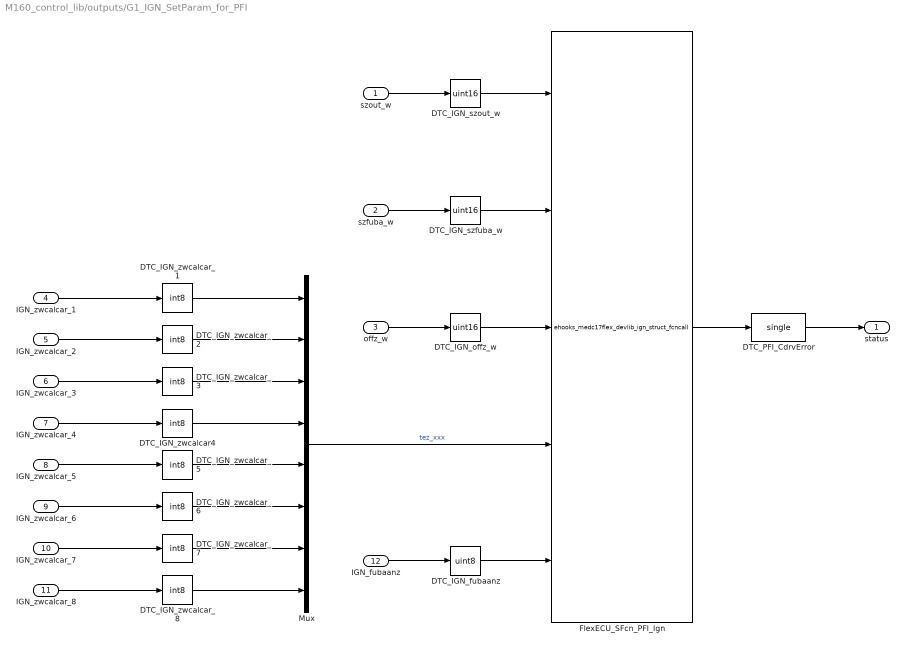
== system M160_control_lib/outputs/G1_IGN_SetParam_for_PFI ==
  szout_w : Inport
  szfuba_w : Inport  Port=2
  offz_w : Inport  Port=3
  IGN_zwcalcar_1 : Inport  Port=4
  IGN_zwcalcar_2 : Inport  Port=5
  IGN_zwcalcar_3 : Inport  Port=6
  IGN_zwcalcar_4 : Inport  Port=7
  IGN_zwcalcar_5 : Inport  Port=8
  IGN_zwcalcar_6 : Inport  Port=9
  IGN_zwcalcar_7 : Inport  Port=10
  IGN_zwcalcar_8 : Inport  Port=11
  IGN_fubaanz : Inport  Port=12
  DTC_IGN_fubaanz : DataTypeConversion  OutDataTypeStr=uint8  RndMeth=Nearest
  DTC_IGN_offz_w : DataTypeConversion  OutDataTypeStr=uint16  RndMeth=Nearest
  DTC_IGN_szfuba_w : DataTypeConversion  OutDataTypeStr=uint16  RndMeth=Nearest
  DTC_IGN_szout_w : DataTypeConversion  OutDataTypeStr=uint16  RndMeth=Nearest
  DTC_IGN_zwcalcar4 : DataTypeConversion  OutDataTypeStr=int8  RndMeth=Nearest
  DTC_IGN_zwcalcar_{1..3,5..8} (7 alike) : DataTypeConversion  OutDataTypeStr=int8  RndMeth=Nearest
  DTC_PFI_CdrvError : DataTypeConversion  OutDataTypeStr=single
  FlexECU_SFcn_PFI_Ign : S-Function  FunctionName=ehooks_medc17flex_devlib_ign_struct_fcncall  Parameters=NoInputPorts, NoOutputPorts, InputPortDataTypes, OutputPortDataTypes, CFunctionArgTypes, CFunctionName, StructMemberNames, StructTypeName, InputPortDataWidths, OutputPortDataWidths  EnableBusSupport=off  mask{NoInputPorts=5, NoOutputPorts=1, InputPortDataTypes=uint16, uint16, uint16, int8,uint8, OutputPortDataTypes=uint8, CFunctionArgTypes=ret,val, val, val, refin, val, CFunctionName=IgnCl_PfiSetParam, StructMemberNames=szout_w, szfuba_w, offz_w, zwcalcar, fubaanz, StructTypeName=IgnClInterface_type, InputPortDataWidths=1,1,1,8,1, OutputPortDataWidths=1}
      mask prompts: NoInputPorts "Number of input ports"; NoOutputPorts "Number of output ports"; InputPortDataTypes "Input port data types"; OutputPortDataTypes "Output port data types"; CFunctionArgTypes "C function argument types"; CFunctionName "C function name"; StructMemberNames "Structure member names"; StructTypeName "Structure type name"; InputPortDataWidths "Input port widths"; OutputPortDataWidths "Output port widths"
      mask Display: disp('EHOOKS FlexECU\nDevLib Wrapper\nS-Function')
  Mux : Mux  Inputs=8
  status : Outport
  wires:
  DTC_PFI_CdrvError/1 -> status/1
  FlexECU_SFcn_PFI_Ign/1 -> DTC_PFI_CdrvError/1
  DTC_IGN_offz_w/1 -> FlexECU_SFcn_PFI_Ign/3
  szout_w/1 -> DTC_IGN_szout_w/1
  DTC_IGN_zwcalcar_1/1 -> Mux/1
  Mux/1 -> FlexECU_SFcn_PFI_Ign/4  "tez_xxx"
  szfuba_w/1 -> DTC_IGN_szfuba_w/1
  DTC_IGN_szfuba_w/1 -> FlexECU_SFcn_PFI_Ign/2
  offz_w/1 -> DTC_IGN_offz_w/1
  IGN_zwcalcar_1/1 -> DTC_IGN_zwcalcar_1/1
  DTC_IGN_fubaanz/1 -> FlexECU_SFcn_PFI_Ign/5
  DTC_IGN_zwcalcar_2/1 -> Mux/2
  IGN_zwcalcar_2/1 -> DTC_IGN_zwcalcar_2/1
  DTC_IGN_zwcalcar_3/1 -> Mux/3
  IGN_zwcalcar_3/1 -> DTC_IGN_zwcalcar_3/1
  DTC_IGN_zwcalcar4/1 -> Mux/4
  IGN_zwcalcar_4/1 -> DTC_IGN_zwcalcar4/1
  DTC_IGN_zwcalcar_5/1 -> Mux/5
  IGN_zwcalcar_5/1 -> DTC_IGN_zwcalcar_5/1
  DTC_IGN_zwcalcar_6/1 -> Mux/6
  IGN_zwcalcar_6/1 -> DTC_IGN_zwcalcar_6/1
  DTC_IGN_zwcalcar_7/1 -> Mux/7
  IGN_zwcalcar_7/1 -> DTC_IGN_zwcalcar_7/1
  DTC_IGN_zwcalcar_8/1 -> Mux/8
  IGN_zwcalcar_8/1 -> DTC_IGN_zwcalcar_8/1
  IGN_fubaanz/1 -> DTC_IGN_fubaanz/1
  DTC_IGN_szout_w/1 -> FlexECU_SFcn_PFI_Ign/1
